simulink model "DualActiveBridgePlant_CurrentCnt"  (R2022a)
settings: Solver=ode23t  StartTime=0.0  StopTime=0.1  FixedStep=Tsw/1000  MaxStep=Tsw/50  RelTol=1e-3  AbsTol=1e-3
PreLoadFcn:
  | DAB_DesignSheet
undefined symbols (not defined in the file): p, Tlpf, Tsw
libraries: slpidlib x1, fl_lib x1, ee_lib x1, nesl_utility x1
settings Model: SimulationMode=rapid-accelerator  Creator=ykamatan  LastModifiedBy=ykamatan
settings SolverCC: AutoScaleAbsTol=off  AlgebraicLoopSolver=TrustRegion
settings DebuggingCC: UnconnectedInputMsg=warning  UnconnectedOutputMsg=warning  UnconnectedLineMsg=warning  SymbolicDimsDataTypeCodeGenerationDiagnostic=none  SFMachineParentedDataDiag=warning
settings SFSimCC: CustomCodeUndefinedFunction=UseInterfaceOnly
settings RTWCC: DLArmComputeVersion=19.05
settings SimscapeCC: SimscapeLogType=local  SimscapeLogSimulationStatistics=on  SimscapeLogToSDI=on  SimscapeLogLimitData=off  SimscapeLogDataHistory=10000

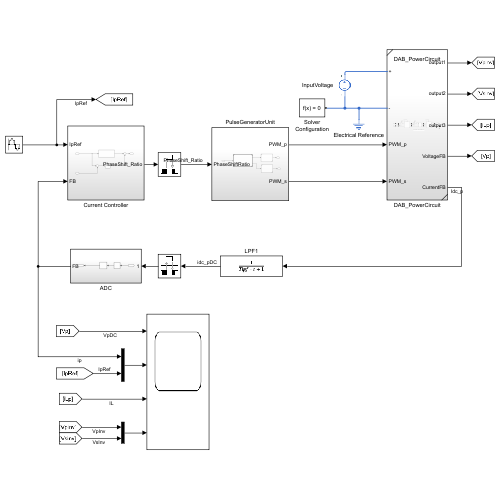
[thumbnail: Simulink's stored preview of the top-level diagram]
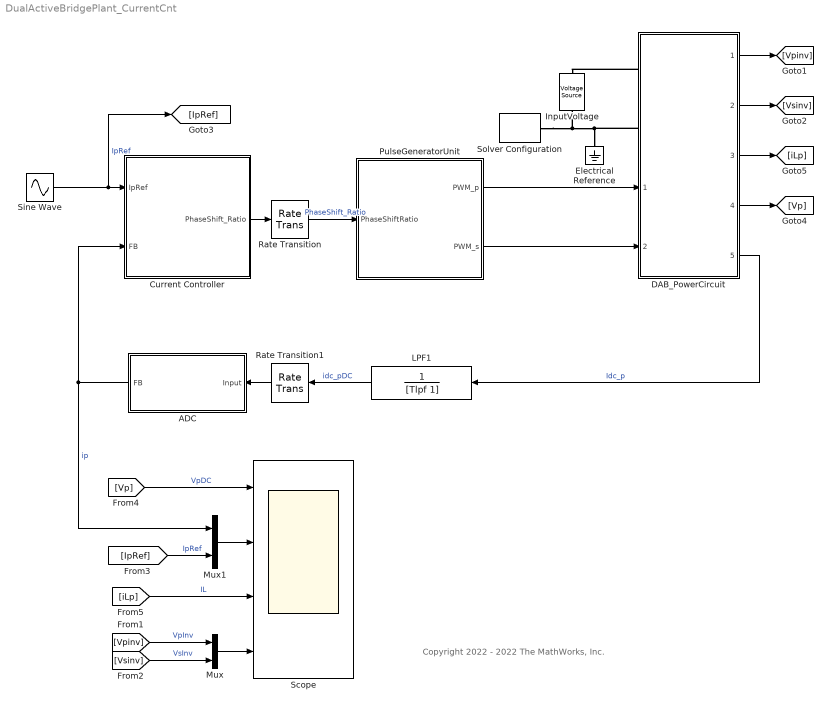
== system DualActiveBridgePlant_CurrentCnt ==
  note: Copyright 2022 - 2022 The MathWorks, Inc.
  ADC : Subsystem
  Current Controller : Subsystem
  DAB_PowerCircuit : Subsystem  ReferencedSubsystem=DAB_PowerCircuit
      settings: PortSchema="{\"entries\":[{\"content\":{\"sides\":[{\"content\":{\"connectorIds\":[\"LConn1\",\"LConn2\",\"In1\",\"In2\"]},\"type\":\"ConnectorPlacement.EquallySpacedRectSide\",\"uuid\":\"828afb30-019f-4264-8411-bc10d9e5858c\"},{\"content\":{\"connectorIds\":[\"Out1\",\"Out2\",\"Out3\",\"Out4\",\"Out5\"],\"side\":\"RIGHT\"},\"type\":\"ConnectorPlacement.EquallySpacedRectSide\",\"uuid\":\"a5597028-647d-41f2-8613-0737d9d532dd\"},{\"content\":{\"connectorIds\":[],\"side\":\"TOP\"},\"type\":\"ConnectorPlacement.EquallySpacedRectSide\",\"uuid\":\"63db0c14-b0cf-4af7-b0f6-89f3f0342ca0\"},{\"content\":{\"connectorIds\":[],\"side\":\"BOTTOM\"},\"type\":\"ConnectorPlacement.EquallySpacedRectSide\",\"uuid\":\"8271aac7-9cea-425f-8ea3-bca48cddb024\"}]},\"type\":\"ConnectorPlacement.EquallySpacedConnector\",\"uuid\":\"a2e479ac-6dd7-4178-b592-9d059eb37ee2\"}],\"packageUris\":[\"http://schema.mathworks.com/mf0/Connector/R2020b\"],\"version\":\"1.0\"}"
  Electrical Reference : fl_lib/Electrical/Electrical Elements/Electrical Reference
      settings: SourceProductBaseCode=PW,SS,VE
  InputVoltage : ee_lib/Sources/Voltage Source  dc_voltage=Vin V  ac_voltage=0 V  ac_shift=0 rad  ac_frequency=60 Hz  noise_mode=0  PSD=0 V^2/Hz  repeatability=1  auto_seed=2619078890  user_seed=0  sample_time=1e-3 s  i_specify=off  i_priority=None  i=0 A  i_nominal_specify=off  i_nominal_unit=A  i_nominal_value=1  v_specify=off  v_priority=None  v=0 V  v_nominal_specify=off  v_nominal_unit=V  v_nominal_value=1
  LPF1 : TransferFcn  Denominator=[Tlpf 1]
  Mux : Mux  Inputs=2
  Mux1 : Mux  Inputs=2
  PulseGeneratorUnit : Subsystem
      settings: PortSchema="{\"entries\":[{\"content\":{\"sides\":[{\"content\":{\"connectorIds\":[\"Out1\",\"Out2\"]},\"type\":\"ConnectorPlacement.EquallySpacedRectSide\",\"uuid\":\"bf5681da-ba91-491c-aae3-0e02de7e88a9\"},{\"content\":{\"connectorIds\":[\"In1\"],\"side\":\"RIGHT\"},\"type\":\"ConnectorPlacement.EquallySpacedRectSide\",\"uuid\":\"1c7570ff-58cb-485b-80f3-8038d236ae35\"},{\"content\":{\"connectorIds\":[],\"side\":\"TOP\"},\"type\":\"ConnectorPlacement.EquallySpacedRectSide\",\"uuid\":\"1d01cce1-4380-4534-925e-d3b589f82d95\"},{\"content\":{\"connectorIds\":[],\"side\":\"BOTTOM\"},\"type\":\"ConnectorPlacement.EquallySpacedRectSide\",\"uuid\":\"ff6b62c9-adc6-469a-b009-d7e5eefa0c45\"}]},\"type\":\"ConnectorPlacement.EquallySpacedConnector\",\"uuid\":\"27e4c4b0-3ff3-438f-a178-d8c4ed4034d3\"}],\"packageUris\":[\"http://schema.mathworks.com/mf0/Connector/R2020b\"],\"version\":\"1.0\"}"
  Rate Transition : RateTransition
  Rate Transition1 : RateTransition
  Scope : Scope  NumInputPorts=4
  Sine Wave : Sin  Amplitude=8  Frequency=2*pi*20  SampleTime=Tsw
  Solver Configuration : nesl_utility/Solver Configuration  PhysicalDomain=network_engine_domain  SubClassName=solver  LeftPortType=input  RightPortType=generic  Tones=[]  Harmonics=[]  SimulateNoise=off  Profile=off  UseLocalSampling=off  EnableSwitchedLinearOptims=on  FrequencyDomain=off  UseCCode=off  RelTol=0.001  AbsTol=1e-06  MinStep=1e-09  ToWorkspace=off  RevertToSquareIcSolve=off  NumHomotopyIterations=100  PhasorMode=off  PhasorModeNumHarmonics=1  IndexReductionMethod=DerivativeReplacement  DoDC=off  ResidualTolerance=1e-09  UseLocalSolver=off  LocalSolverChoice=NE_BACKWARD_EULER_ADVANCER  LocalSolverSampleTime=0.001  DoFixedCost=off  MaxNonlinIter=3  MaxModeIter=2  ComputeImpulses=off  ImpulseIterations=2  LinearAlgebra=auto  LinearAlgebraNumThread=0  EquationFormulation=NE_TIME_EF  DelaysMemoryBudget=1024  AutomaticFiltering=on  FilteringTimeConstant=0.001  PartitionStorageMethod=AS_NEEDED  PartitionMemoryBudget=1024  PartitionMethod=ROBUST
      settings: SourceProductBaseCode=SS,PW,VE
  wires:
  Rate Transition/1 -> PulseGeneratorUnit/1(PhaseShiftRatio)  "PhaseShift_Ratio"
  Mux1/1 -> Scope/2
  [Vpinv] -> Mux/1  "VpInv"
  DAB_PowerCircuit/5 -> LPF1/1  "Idc_p"
  [iLp] -> Scope/3  "IL"
  Mux/1 -> Scope/4
  [Vsinv] -> Mux/2  "VsInv"
  Sine Wave/1 -> Current Controller/1(IpRef), [IpRef]  "IpRef"
  [IpRef] -> Mux1/2  "IpRef"
  [Vp] -> Scope/1  "VpDC"
  LPF1/1 -> Rate Transition1/1  "idc_pDC"
  Current Controller/1(PhaseShift_Ratio) -> Rate Transition/1
  PulseGeneratorUnit/2(PWM_p) -> DAB_PowerCircuit/1
  PulseGeneratorUnit/1(PWM_s) -> DAB_PowerCircuit/2
  DAB_PowerCircuit/1 -> [Vpinv]
  DAB_PowerCircuit/2 -> [Vsinv]
  DAB_PowerCircuit/4 -> [Vp]
  ADC/1(FB) -> Mux1/1, Current Controller/2(FB)  "ip"
  Rate Transition1/1 -> ADC/1(Input)
  DAB_PowerCircuit/3 -> [iLp]
  connections:
  DAB_PowerCircuit/LConn1 -- InputVoltage/LConn1
  Solver Configuration/RConn1 -- InputVoltage/RConn1 -- DAB_PowerCircuit/LConn2 -- Electrical Reference/LConn1

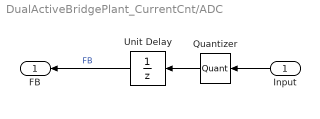
== system DualActiveBridgePlant_CurrentCnt/ADC ==
  Input : Inport
  Quantizer : Quantizer  QuantizationInterval=0.01
  Unit Delay : UnitDelay  SampleTime=Tsw  HasFrameUpgradeWarning=on
  FB : Outport
  wires:
  Quantizer/1 -> Unit Delay/1
  Unit Delay/1 -> FB/1  "FB"
  Input/1 -> Quantizer/1

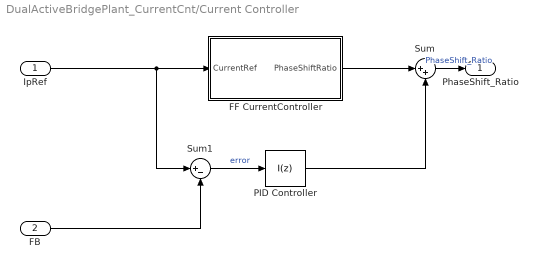
== system DualActiveBridgePlant_CurrentCnt/Current Controller ==
  IpRef : Inport
  FB : Inport  Port=2
  FF CurrentController : Subsystem
  PID Controller : slpidlib/PID Controller  Controller=I  Form=Parallel  TimeDomain=Discrete-time  UseExternalTs=off  SampleTime=Tsw  IntegratorMethod=Forward Euler  FilterMethod=Forward Euler  ControllerParametersSource=internal  P=0.1  I=10  UseKiTs=off  D=0  N=100  UseFilter=on  TunerSelectOption=Transfer Function Based (PID Tuner App)  InitialConditionSource=internal  InitialConditionForIntegrator=0  InitialConditionForFilter=0  DifferentiatorICPrevScaledInput=0  ExternalReset=none  TrackingMode=off  Kt=1  LimitOutput=off  SatLimitsSource=internal  UpperSaturationLimit=inf  LowerSaturationLimit=-inf  LinearizeAsGain=on  AntiWindupMode=none  Kb=1  POutMin=[]  POutMax=[]  IOutMin=[]  IOutMax=[]  DOutMin=[]  DOutMax=[]  NOutMin=[]  NOutMax=[]  SumOutMin=[]  SumOutMax=[]  SaturationOutMin=[]  SaturationOutMax=[]  PParamMin=[]  PParamMax=[]  IParamMin=[]  IParamMax=[]  DParamMin=[]  DParamMax=[]  NParamMin=[]  NParamMax=[]  KbParamMin=[]  KbParamMax=[]  KtParamMin=[]  KtParamMax=[]  KbOutMin=[]  KbOutMax=[]  KtOutMin=[]  KtOutMax=[]  IntegratorOutMin=[]  IntegratorOutMax=[]  FilterOutMin=[]  FilterOutMax=[]  SumI1OutMin=[]  SumI1OutMax=[]  SumI2OutMin=[]  SumI2OutMax=[]  SumI3OutMin=[]  SumI3OutMax=[]  SumI4OutMin=[]  SumI4OutMax=[]  SumDOutMin=[]  SumDOutMax=[]  DifferentiatorOutMin=[]  DifferentiatorOutMax=[]  FilterDiffOutCoefMin=[]  FilterDiffOutCoefMax=[]  ReciprocalOutMin=[]  ReciprocalOutMax=[]  SumDenOutMin=[]  SumDenOutMax=[]  SumNumOutMin=[]  SumNumOutMax=[]  DivideOutMin=[]  DivideOutMax=[]  UdiffTsProdOutMin=[]  UdiffTsProdOutMax=[]  NTsProdOutMin=[]  NTsProdOutMax=[]  UintegralTsProdOutMin=[]  UintegralTsProdOutMax=[]  UngainTsProdOutMin=[]  UngainTsProdOutMax=[]  IntegratorContinuousStateAttributes=''  IntegratorStateMustResolveToSignalObject=off  IntegratorRTWStateStorageClass=Auto  FilterContinuousStateAttributes=''  FilterStateMustResolveToSignalObject=off  FilterRTWStateStorageClass=Auto  ParallelPVariant=Disabled  IdealPVariant=Disabled  IVariant=InternalParameters  DVariant=Disabled  IntegratorVariant=Discrete  SatVariant=Disabled  AWVariant=Passthrough  PCopyVariant=Disabled  TRVariant=Disabled  FdbkBlocksVariant=Forward  IdealPFdbkVariant=Disabled  SatFdbkVariant=Disabled  DerivativeFilterVariant=Disabled  NVariant=Disabled  NCopyVariant=Disabled_SignalSpec  FilterICVariant=Disabled  IntegratorICVariant=InternalICs  ExternalResetVariant=Disabled  TRSumVariant=Passthrough  SumFdbkVariant=Disabled  SumVariant=Passthrough_I  TsampFilterVariant=InternalTs  TsampNgainVariant=Passthrough  TsampIntegralVariant=Passthrough  ExternalSaturationOutDataTypeStr=Inherit: Same as second input  aMode=0
  Sum : Sum  Inputs=|++
  Sum1 : Sum  Inputs=|+-
  PhaseShift_Ratio : Outport
  wires:
  FF CurrentController/1(PhaseShiftRatio) -> Sum/1
  IpRef/1 -> FF CurrentController/1(CurrentRef), Sum1/1
  Sum1/1 -> PID Controller/1  "error"
  FB/1 -> Sum1/2
  PID Controller/1 -> Sum/2
  Sum/1 -> PhaseShift_Ratio/1  "PhaseShift_Ratio"

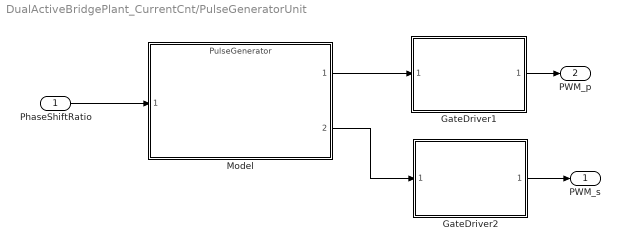
== system DualActiveBridgePlant_CurrentCnt/PulseGeneratorUnit ==
  PhaseShiftRatio : Inport
  GateDriver1 : Subsystem  ReferencedSubsystem=GateDriver
      settings: PortSchema="{\"entries\":[{\"content\":{\"sides\":[{\"content\":{\"connectorIds\":[\"Out1\"]},\"type\":\"ConnectorPlacement.EquallySpacedRectSide\",\"uuid\":\"311475b7-00eb-40fb-907f-61918164ee7b\"},{\"content\":{\"connectorIds\":[\"In1\"],\"side\":\"RIGHT\"},\"type\":\"ConnectorPlacement.EquallySpacedRectSide\",\"uuid\":\"0b8731f7-8da9-403f-8880-992b54f942ab\"},{\"content\":{\"connectorIds\":[],\"side\":\"TOP\"},\"type\":\"ConnectorPlacement.EquallySpacedRectSide\",\"uuid\":\"6fd0a64f-df87-43d4-a7cc-9e3ddd37bd1a\"}]},\"type\":\"ConnectorPlacement.EquallySpacedConnector\",\"uuid\":\"c1f4b631-9d66-4028-87ab-7567590c1b71\"}],\"packageUris\":[\"http://schema.mathworks.com/mf0/Connector/R2020b\"],\"version\":\"1.0\"}"
  GateDriver2 : Subsystem  ReferencedSubsystem=GateDriver
  Model : ModelReference  ModelNameDialog=PulseGenerator.slx  SimulationMode=Normal  ModelReferenceVersion=5.0
  PWM_s : Outport
  PWM_p : Outport  Port=2
  wires:
  GateDriver2/1 -> PWM_s/1
  PhaseShiftRatio/1 -> Model/1
  Model/2 -> GateDriver2/1
  Model/1 -> GateDriver1/1
  GateDriver1/1 -> PWM_p/1

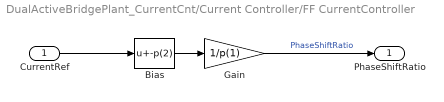
== system DualActiveBridgePlant_CurrentCnt/Current Controller/FF CurrentController ==
  CurrentRef : Inport
  Bias : Bias  Bias=-p(2)  SaturateOnIntegerOverflow=off
  Gain : Gain  Gain=1/p(1)
  PhaseShiftRatio : Outport
  wires:
  Bias/1 -> Gain/1
  Gain/1 -> PhaseShiftRatio/1  "PhaseShiftRatio"
  CurrentRef/1 -> Bias/1
